simulink model "khallivalli"  (R2017b)
settings: Solver=VariableStepAuto  StartTime=0.0  StopTime=10.0  RelTol=1e-3
values from neighbouring files (symbols this model uses):
  xq = max(min(xq, 2^15-1), -2^15)    [convert_audio_coe.m]
libraries: xbsIndex_r4 x6
settings Model: Creator=8183302  LastModifiedBy=8183302

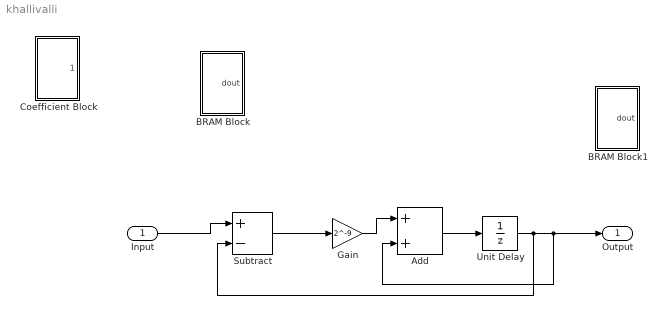
== system khallivalli ==
  Input : Inport
  Add : Sum
  BRAM Block : Subsystem
  BRAM Block1 : Subsystem
  Coefficient Block : Subsystem
  Gain : Gain  Gain=2^-9
  Subtract : Sum  Inputs=+-
  Unit Delay : UnitDelay  SampleTime=-1
  Output : Outport
  wires:
  Gain/1 -> Add/1
  Input/1 -> Subtract/1
  Unit Delay/1 -> Add/2, Output/1, Subtract/2
  Add/1 -> Unit Delay/1
  Subtract/1 -> Gain/1

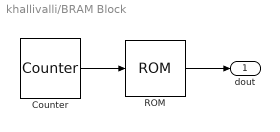
== system khallivalli/BRAM Block ==
  Counter : xbsIndex_r4/Counter  cnt_type=Count Limited  cnt_to=length(xq)-1  operation=Up  start_count=0  cnt_by_val=1  arith_type=Unsigned  n_bits=ceil(log2(length(xq)))  bin_pt=0  load_pin=off  rst=off  en=off  explicit_period=on  period=1  use_behavioral_HDL=off  implementation=Fabric  dbl_ovrd=off  block_type=counter
  ROM : xbsIndex_r4/ROM  depth=length(xq)  initVector=test.coe  distributed_mem=Block RAM  rst=off  init_reg=0  en=off  latency=1  gui_display_data_type=Fixed-point  arith_type="Signed  (2's comp)"  n_bits=16  bin_pt=14  preci_type=Single  exp_width=8  frac_width=24  optimize=Area  use_rpm=on  dbl_ovrd=off  block_type=sprom
  dout : Outport
  wires:
  ROM/1 -> dout/1
  Counter/1 -> ROM/1

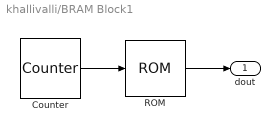
== system khallivalli/BRAM Block1 ==
  Counter : xbsIndex_r4/Counter  cnt_type=Count Limited  cnt_to=length(xq)-1  operation=Up  start_count=0  cnt_by_val=1  arith_type=Unsigned  n_bits=ceil(log2(length(xq)))  bin_pt=0  load_pin=off  rst=off  en=off  explicit_period=on  period=1  use_behavioral_HDL=off  implementation=Fabric  dbl_ovrd=off  block_type=counter
  ROM : xbsIndex_r4/ROM  depth=length(xq)  initVector=test.coe  distributed_mem=Block RAM  rst=off  init_reg=0  en=off  latency=1  gui_display_data_type=Fixed-point  arith_type="Signed  (2's comp)"  n_bits=16  bin_pt=15  preci_type=Single  exp_width=8  frac_width=24  optimize=Area  use_rpm=on  dbl_ovrd=off  block_type=sprom
  dout : Outport
  wires:
  ROM/1 -> dout/1
  Counter/1 -> ROM/1

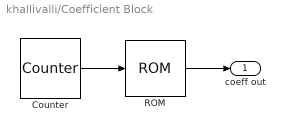
== system khallivalli/Coefficient Block ==
  Counter : xbsIndex_r4/Counter  cnt_type=Count Limited  cnt_to=159  operation=Up  start_count=0  cnt_by_val=1  arith_type=Unsigned  n_bits=8  bin_pt=0  load_pin=off  rst=off  en=off  explicit_period=on  period=1  use_behavioral_HDL=off  implementation=Fabric  dbl_ovrd=off  block_type=counter
  ROM : xbsIndex_r4/ROM  depth=160  initVector=coeff.coe  distributed_mem=Block RAM  rst=off  init_reg=0  en=off  latency=1  gui_display_data_type=Fixed-point  arith_type="Signed  (2's comp)"  n_bits=16  bin_pt=14  preci_type=Single  exp_width=8  frac_width=24  optimize=Area  use_rpm=on  dbl_ovrd=off  block_type=sprom
  coeff out : Outport
  wires:
  ROM/1 -> coeff out/1
  Counter/1 -> ROM/1
